simulink model "Uebung_matlabtest"  (R2017b)
settings: Solver=ode45  StartTime=0.0  StopTime=50  MaxStep=1e-3  RelTol=1e-3
settings Model: Creator=lukasschwoerer  LastModifiedBy=lukasschwoerer

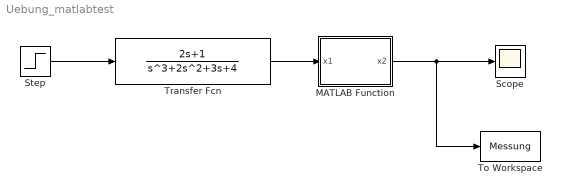
== system Uebung_matlabtest ==
  MATLAB Function : MATLAB Function  TreatAsAtomicUnit=on
  Scope : Scope
  Step : Step  SampleTime=0
  To Workspace : ToWorkspace  VariableName=Messung  SaveFormat=Structure With Time  SampleTime=-1
  Transfer Fcn : TransferFcn  Numerator=[2 1]  Denominator=[1 2 3 4]
  wires:
  Step/1 -> Transfer Fcn/1
  Transfer Fcn/1 -> MATLAB Function/1(x1)
  MATLAB Function/1(x2) -> To Workspace/1, Scope/1

== matlab function Uebung_matlabtest/MATLAB Function ==
  data: x1 input; x2 output
function x2 = fcn(x1)
if x1<=0
    x2=0;
else
    if x1>=2
        x2 = 0;
    else
        x2 = 2*sin(pi*x1);
        
    end
end
end
